simulink model "TissueModel1_linear"  (R2016a)
settings: Solver=ode3  StartTime=0.0  StopTime=tend  FixedStep=1e-3  MaxStep=0.1  RelTol=1e-3
values from neighbouring files (symbols this model uses):
  phi = paramsPatient{gg} + randn(1,key.paramsize).*paramNoise    [CreateSimData.m]    (also in CreateSimDataLocations.m = paramBase + randn(1,key.paramsize).*paramNoise; testExponentials.m = 2; test_LinearLeastSquares.m = pinv(dtemp)*utemp; test_NonLinearModel.m = paramrefine([2,3,4]))
undefined symbols (not defined in the file or in its folder): psi
settings Model: Creator=pjseiler  LastModifiedBy=rod
settings DataIOCC: LimitDataPoints=on  SaveFormat=Array  SignalLoggingSaveFormat=ModelDataLogs
settings OptimizationCC: ExpressionDepthLimit=2147483647
settings DebuggingCC: UnderspecifiedInitializationDetection=Classic  MergeDetectMultiDrivingBlocksExec=none  SolverPrmCheckMsg=warning  MultiTaskDSMMsg=warning  MultiTaskCondExecSysMsg=none  FcnCallInpInsideContextMsg=EnableAllAsWarning  StateNameClashWarn=warning
settings HardwareCC: ProdBitPerPointer=32  ProdLargestAtomicFloat=None  ProdIntDivRoundTo=Undefined  ProdEndianess=Unspecified  ProdWordSize=32  ProdHWDeviceType=32-bit Generic
settings ModelReferenceCC: PropagateSignalLabelsOutOfModel=off
settings GRTTargetCC: CombineOutputUpdateFcns=off  GRTInterface=on
settings ConfigComp: CovModelRefEnable=Off

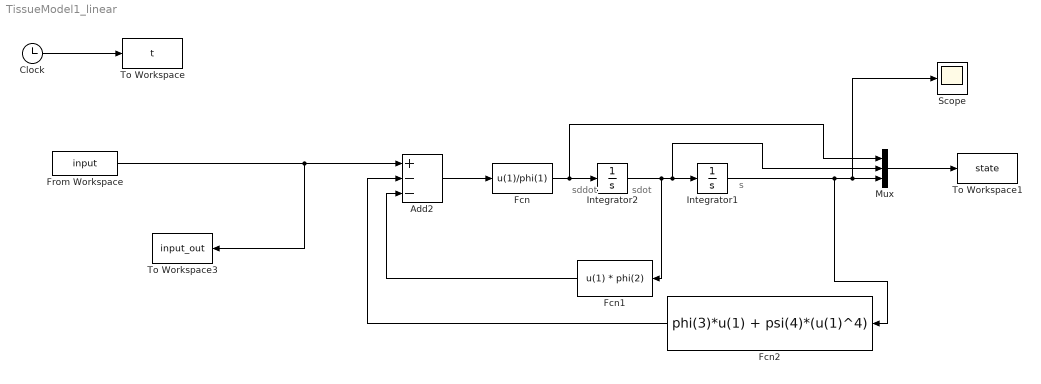
== system TissueModel1_linear ==
  note: sddot
  note: sdot
  note: s
  Add2 : Sum  Inputs=+--
  Clock : Clock
  Fcn : Fcn  Expr=u(1)/phi(1)
  Fcn1 : Fcn  Expr=u(1) * phi(2)
  Fcn2 : Fcn  Expr=phi(3)*u(1) + psi(4)*(u(1)^4)
  From Workspace : FromWorkspace  VariableName=input  SampleTime=0
  Integrator1 : Integrator
  Integrator2 : Integrator
  Mux : Mux  Inputs=3
  Scope : Scope
  To Workspace : ToWorkspace  VariableName=t  SampleTime=-1
  To Workspace1 : ToWorkspace  VariableName=state  SaveFormat=Timeseries  SampleTime=-1
  To Workspace3 : ToWorkspace  VariableName=input_out  SaveFormat=Timeseries  SampleTime=-1
  wires:
  Clock/1 -> To Workspace/1
  Integrator2/1 -> Fcn1/1, Integrator1/1, Mux/2
  Integrator1/1 -> Fcn2/1, Mux/3, Scope/1
  Add2/1 -> Fcn/1
  Fcn1/1 -> Add2/3
  Fcn2/1 -> Add2/2
  Mux/1 -> To Workspace1/1
  From Workspace/1 -> Add2/1, To Workspace3/1
  Fcn/1 -> Mux/1, Integrator2/1
